simulink model "segway_torque_control"  (R2022a)
settings: Solver=FixedStepAuto  StartTime=0.0  StopTime=10  FixedStep=1e-3  RelTol=1e-3
PreLoadFcn:
  | preload
InitFcn:
  | init
  | preload
values from neighbouring files (symbols this model uses):
  A1 = [0 0   1 0 ... (first row only)    [plant.m]
  A2 = [0   1 ... (first row only)    [plant.m]
  alpha = n * Kt    [plant.m]
  B1 = [0 0 ... (first row only)    [plant.m]
  B2 = [0    0 ... (first row only)    [plant.m]
  C1 = [1 0 0 0 ... (first row only)    [plant.m]
  C2 = [1 0 ... (first row only)    [plant.m]
  chi0 = zeros(N_ukf, 2*N_ukf+1)    [UKF_params.m]
  D = 0.2    [params.m]
  D1 = zeros(4, 2)    [plant.m]
  D2 = zeros(2)    [plant.m]
  Fd = sysd.A    [LKF_params.m]
  fm = evalin('base', 'fm')    [f.m]    (also in params.m = 0.0022)
  fw = 0.0    (= 0)    [params.m]
  g = 9.81    [params.m]
  Gd = sysd.B    [LKF_params.m]
  h = 0.39    [params.m]
  H_ekf = [0 1 0 0 0 0 0 ... (first row only)    [EKF_params.m]
  H_lkf = [0 1 0 0 0 0 0 ... (first row only)    [LKF_params.m]
  H_ukf = [0 1 0 0 0 0 0 ... (first row only)    [UKF_params.m]
  Jm = 1e-5    (= 1e-05)    [params.m]
  Jphi = M * (W^2 + D^2) / 12    (= 0.126774333333)    [params.m]
  Jpsi = M * L^2 / 3    (= 0.08910525)    [params.m]
  Jw = m * R^2 / 2    (= 0.01146068)    [params.m]
  Jwx = m * (3*R^2 + hw^2) / 12    (= 0.00610456)    [params.m]
  K_lqr = lqrd(s4.A, s4.B, QQ, RR, Ts)    [control.m]
  Kt = 2.28    [params.m]
  L = h / 2    (= 0.195)    [params.m]
  lambda_ukf = alpha_ukf^2 * (N_ukf + kappa_ukf) - N_ukf    [UKF_params.m]
  M = 7.03    [params.m]
  m = 1.54    [params.m]
  n = 1    [params.m]
  N_ukf = length(x0_ukf)    [UKF_params.m]
  P0_ekf = eye(7)*0.1    [EKF_params.m]
  P0_lkf = eye(7)*0.1    [LKF_params.m]
  P0_ukf = eye(7)*0.1    [UKF_params.m]
  Q_ekf = [0.1*Ts^4/4     Ts^3/2     0          Ts^2/2     0          0          0 ... (first row only)    [EKF_params.m]
  Q_lkf = [Ts^4/4     Ts^3/2     0          Ts^2/2     0          0          0 ... (first row only)    [LKF_params.m]
  Q_ukf = [0.0025*Ts^4 Ts^3/2     0          Ts^2/2     0          0          0 ... (first row only)    [UKF_params.m]
  R = 0.122    [params.m]
  R_ekf = [sigma_y_ekf(1) 0          0          0          0 ... (first row only)    [EKF_params.m]
  R_lkf = [sigma_y(1) 0          0          0          0 ... (first row only)    [LKF_params.m]
  R_ukf = [sigma_y_ukf(1) 0          0          0          0 ... (first row only)    [UKF_params.m]
  Ts = 0.01    [params.m]
  W = 0.42    [params.m]
  w_c_ukf = diag(wi*ones([1, 2*N_ukf+1]))    [UKF_params.m]
  w_m_ukf = wi*ones([1, 2*N_ukf+1])    [UKF_params.m]
  x0_ekf = [0; 0; 0; 0; 0; 0; 0]    [EKF_params.m]
  x0_lkf = [0; 0; 0; 0; 0; 0; 0]    [LKF_params.m]
  x0_ukf = [0; 0; 0; 0; 0; 0; 0]    [UKF_params.m]
  Z0_ukf = zeros(5, 2*N_ukf+1)    [UKF_params.m]
undefined symbols (not defined in the file or in its folder): X, Y, Z
libraries: sm_lib x18, nesl_utility x14, simulink_extras x4, simulink x1
(part 2 of 2)

== stateflow chart segway_torque_control/UKF ==
  state Predict
    %----------------------------------------------
    %PREDICT
    % sigma transform
    chi(:,1) = x_hat;
    L_sqrt = chol((N_ukf + lambda_ukf)*P);
    for i = 2:(2*N_ukf+1)
    if i <= (N_ukf+1)
    chi(:,i) = x_hat + L_sqrt(:,i-1);
    else
    chi(:,i) = x_hat - L_sqrt(:,i-N_ukf-1);
    end
    end
    % propagation through non-linear funtion
    for i = 1:(2*N_ukf+1)
    chi_(:,i) = dynamics(chi(:,i), u, n ,fm, Kt, fw, m, M, L, R, W, Ts, Jm, Jw, Jpsi, Jphi, g);
    end
    % mean and covariance computation
    x_hat_ = chi_ * w_m_ukf.';
    P_ = (chi_ - x_hat_) * w_c_ukf * (chi_ - x_hat_).' + Q_ukf;
    %----------------------------------------------
    %UPDATE
    % propagate through obsevation matrix
    for i = 1:(2*N_ukf+1)
    Z(:,i) = H_ukf * chi_(:,i);
    end
    % mean and cross-covariance computation
    mu_z = Z * w_m_ukf.';
    Pz = (Z - mu_z) * w_c_ukf * (Z - mu_z).' + R_ukf;
    Pxz = (chi_ - x_hat_) * w_c_ukf * (Z - mu_z).';
    % Kalman Gain computation
    K_ukf = Pxz * inv(Pz);
    % estimate state and new covariance
    x_hat = x_hat_ + K_ukf * (y - mu_z);
    %P_
    %K_ukf
    %Pz
    P = P_ - K_ukf * Pz * K_ukf.';
    %----------------------------------------------
  (default) -> Predict : {x_hat = x0_ukf; P = P0_ukf; chi = chi0; chi_ = chi0; Z = Z0_ukf;}
  data: x function_input; u_ function_input; state function_output; n_ function_input; fm_ function_input; Kt_ function_input; fw_ function_input; m_ function_input; M_ function_input; L_ function_input; R_ function_input; W_ function_input; Ts_ function_input; Jm_ function_input; Jw_ function_input; Jpsi_ function_input; Jphi_ function_input; g_ function_input; u input; y input; P local; P_ local; x_ local; fm parameter; n parameter; Kt parameter; Ts parameter; fw parameter; m parameter; L parameter; M parameter; R parameter; W parameter; x_hat output; Jm parameter; Jpsi parameter; Jw parameter; g parameter; Jphi parameter; N_ukf parameter; P0_ukf parameter; Q_ukf parameter; lambda_ukf parameter; w_c_ukf parameter; w_m_ukf parameter; x0_ukf parameter; L_sqrt local; chi local double; chi_ local double; i local; x_hat_ local; chi0 parameter; H_ukf parameter; Z local; Z0_ukf parameter; mu_z local; R_ukf parameter; Pz local; Pxz local; K_ukf local
  function state = dynamics(x, u_, n_, fm_, Kt_, fw_, m_, M_, L_, R_, W_, Ts_, Jm_, Jw_, Jpsi_, Jphi_, g_):
    | 
    | function state = dynamics(x, u_, n_, fm_, Kt_, fw_, m_, M_, L_, R_, W_, Ts_, Jm_, Jw_, Jpsi_, Jphi_, g_)
    |     alpha = n_*Kt_;
    |     beta = fm_;
    | 
    |     F_11 = 2*(beta+fw_);
    |     F_12 = -beta;
    |     F_21 = -beta;
    |     F_22 = beta;
    | 
    |     E_11 = (2*m_+M_)*R_^2 + 2*Jw_ + 2*n_^2*Jm_;
    |     E_12 = M_*L_*R_ - 2*n_^2*Jm_;
    |     E_21 = E_12;
    |     E_22 = M_*L_^2 + Jpsi_ + 2*n_^2*Jm_;
    |     detE = E_11*E_22 - E_12*E_21;
    | 
    |     I = 0.5*m_*W_^2 + Jphi_ + (W_^2/(2*R_^2))*(Jw_ + n_^2*Jm_);
    |     J = (W_^2/(2*R_^2))*(beta + fw_);
    |     K = (W_/(2*R_))*alpha;
    |     
    | 
    |     eq4 = -E_12*(-F_21*x(4) - F_22*x(5) + L_^2*M_*x(7)^2*sin(x(3))*cos(x(3)) + L_*M_*g_*sin(x(3)) + alpha*(-u_(1) - u_(2)))/detE + E_22*(-F_11*x(4) - F_12*x(5) + L_*M_*R_*x(5)^2*sin(x(3)) + alpha*(u_(1) + u_(2)))/detE;
    |     eq5 = E_11*(-F_21*x(4) - F_22*x(5) + L_^2*M_*x(7)^2*sin(x(3))*cos(x(3)) + L_*M_*g_*sin(x(3)) + alpha*(-u_(1) - u_(2)))/detE - E_21*(-F_11*x(4) - F_12*x(5) + L_*M_*R_*x(5)^2*sin(x(3)) + alpha*(u_(1) + u_(2)))/detE;
    |     eq6 = (-J*x(7) + K*(-u_(1) + u_(2)) - 2*L_^2*M_*x(5)*x(7)*sin(x(3))*cos(x(3)))/I;
    | 
    |     state = [x(1) + x(2)*Ts_; 
    |           x(2) + x(4)*Ts_; 
    |           x(3) + x(5)*Ts_; 
    |           x(4) + eq4*Ts_; 
    |           x(5) + eq5*Ts_; 
    |           x(6) + x(7)*Ts_; 
    |           x(7) + eq6*Ts_];
    | 
    | %     jacobian = eye(7);
    | % 
    | %     jacobian(1,2) = Ts_;
    | %     jacobian(2,4) = Ts_;
    | %     jacobian(3,5) = Ts_;
    | %     jacobian(6,7) = Ts_;
    | %     
    | %     
    | %     jacobian(4,3) = -Ts_*L_*M_*(E_12*(-2*L_*state(7)^2*sin(state(3))^2 + L_*state(7)^2 + g*cos(state(3))) - E_22*R*state(5)^2*cos(state(3)))/detE;
    | %     jacobian(4,4) = (Ts_*(E_12*F_21 - E_22*F_11) + detE)/detE;
    | %     jacobian(4,5) = Ts_*(E_12*F_22 - E_22*(F_12 - 2*L_*M_*R*state(5)*sin(state(3))))/detE;
    | %     jacobian(4,7) = -Ts_*E_12*L_^2*M_*state(7)*sin(2*state(3))/detE;
    | %     jacobian(5,3) = Ts_*L_*M_*(E_11*(-2*L_*state(7)^2*sin(state(3))^2 + L_*state(7)^2 + g*cos(state(3))) - E_21*R*state(5)^2*cos(state(3)))/detE;
    | %     jacobian(5,4) = Ts_*(-E_11*F_21 + E_21*F_11)/detE;
    | %     jacobian(5,5) = (-Ts_*(E_11*F_22 - E_21*(F_12 - 2*L_*M_*R*state(5)*sin(state(3)))) + detE)/detE;
    | %     jacobian(5,7) = Ts_*E_11*L_^2*M_*state(7)*sin(2*state(3))/detE;
    | % 
    | %     jacobian(7,3) = -2*Ts_*L_^2*M_*state(5)*state(7)*cos(2*state(3))/I;
    | %     jacobian(7,5) = -Ts_*L_^2*M_*state(7)*sin(2*state(3))/I;
    | %     jacobian(7,7) = (-Ts_*(J + L_^2*M_*state(5)*sin(2*state(3))) + I)/I;
    | 
    | end
